simulink model "LTI_Output_CHECKED"  (Simulink 8.0)
settings: Solver=ode45  StartTime=0.0  StopTime=10.0  RelTol=1e-3
undefined symbols (not defined in the file or in its folder): Aii, Aij, Bi, Cki, Ckj, D
settings Model: Creator=chepeadan  LastModifiedBy=koehler
settings DataIOCC: SignalLoggingSaveFormat=ModelDataLogs
settings DebuggingCC: FcnCallInpInsideContextMsg=UseLocalSettings  StrictBusMsg=Warning
settings GRTTargetCC: CombineOutputUpdateFcns=off  GRTInterface=on

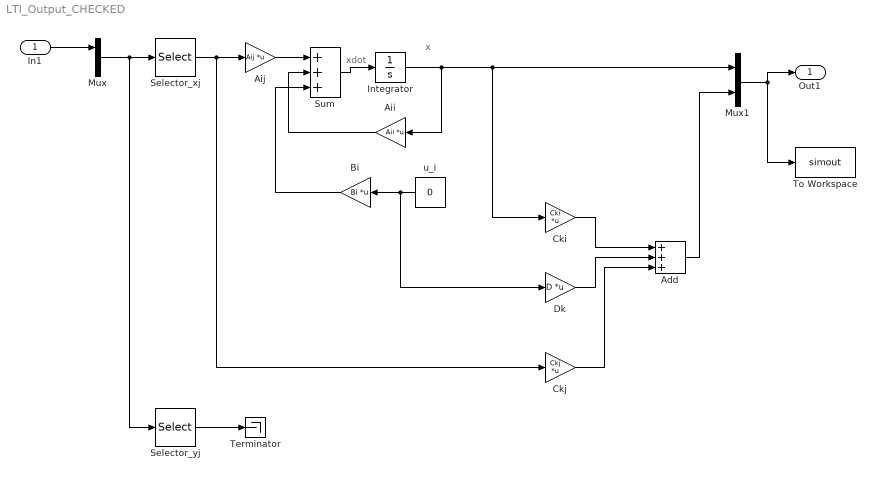
== system LTI_Output_CHECKED ==
  note: xdot
  note: x
  In1 : Inport
  Add : Sum  Inputs=+++
  Aii : Gain  Gain=Aii  Multiplication=Matrix(K*u)
  Aij : Gain  Gain=Aij  Multiplication=Matrix(K*u)
  Bi : Gain  Gain=Bi  Multiplication=Matrix(K*u)
  Cki : Gain  Gain=Cki  Multiplication=Matrix(K*u)
  Ckj : Gain  Gain=Ckj  Multiplication=Matrix(K*u)
  Dk : Gain  Gain=D  Multiplication=Matrix(K*u)
  Integrator : Integrator
  Mux : Mux  Inputs=2
  Mux1 : Mux  Inputs=2
  Selector_xj : Selector  InputPortWidth=2  IndexOptions=Index vector (dialog)  Indices=[1]  OutputSizes=1
  Selector_yj : Selector  InputPortWidth=2  IndexOptions=Index vector (dialog)  Indices=[1]  OutputSizes=1
  Sum : Sum  Inputs=|+|+|+
  Terminator : Terminator
  To Workspace : ToWorkspace  VariableName=simout  SampleTime=-1  SaveFormat=Structure With Time
  u_i : Constant  Value=0
  Out1 : Outport
  wires:
  In1/1 -> Mux/1
  Integrator/1 -> Aii/1, Cki/1, Mux1/1
  Aij/1 -> Sum/1
  Aii/1 -> Sum/2
  u_i/1 -> Dk/1, Bi/1
  Bi/1 -> Sum/3
  Sum/1 -> Integrator/1
  Cki/1 -> Add/1
  Dk/1 -> Add/2
  Add/1 -> Mux1/2
  Mux1/1 -> To Workspace/1, Out1/1
  Ckj/1 -> Add/3
  Mux/1 -> Selector_yj/1, Selector_xj/1
  Selector_xj/1 -> Ckj/1, Aij/1
  Selector_yj/1 -> Terminator/1
